simulink model "interface"  (Simulink 8.5)
settings: Solver=ode45  StartTime=0.0  StopTime=10.0  RelTol=1e-3
settings Model: Creator=GSavaia  LastModifiedBy=GSavaia
settings DataIOCC: SignalLoggingSaveFormat=Dataset
settings OptimizationCC: ExpressionDepthLimit=128
settings DebuggingCC: UnderspecifiedInitializationDetection=Simplified  MergeDetectMultiDrivingBlocksExec=error  FcnCallInpInsideContextMsg=EnableAllAsError  StateNameClashWarn=none
settings GRTTargetCC: CombineOutputUpdateFcns=on  GRTInterface=off

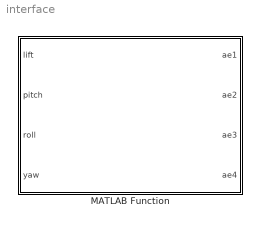
== system interface ==
  MATLAB Function : MATLAB Function  TreatAsAtomicUnit=on

== matlab function MATLAB Function ==
  data: lift input double; ae1 output double; pitch input double; roll input double; yaw input double; ae2 output double; ae3 output double; ae4 output double
function [ae1, ae2, ae3, ae4] = interface(lift, pitch, roll, yaw)

% PARAMETERS
scale_lift = -16400;
scale_pitch = 8240;
scale_roll = 8240;
scale_yaw = 16400;

scales = diag( [scale_pitch, scale_roll, scale_yaw, scale_lift] );
coeff = [+2 +0 -1 -1; ...
         +0 -2 +1 -1; ...
         -2 +0 -1 -1; ...
         +0 +2 +1 -1];
motors = 1/4.*coeff*scales*[pitch;roll;yaw;lift];

motors( motors < 0 ) = 0;

ae1 = sqrt( motors(1) );
ae2 = sqrt( motors(2) );
ae3 = sqrt( motors(3) );
ae4 = sqrt( motors(4) );

end
